simulink library "SUB_ECU_L4_MABX_HW_Interface"  (R2018a)
settings: Solver=VariableStepAuto  StartTime=0.0  StopTime=10.0  RelTol=1e-3
PostLoadFcn:
  | , if any(exist('dsrtsu_mdlpostloadfcn', 'file') == [2, 3, 6]), try dsrtsu_mdlpostloadfcn('Execute', bdroot); catch fprintf('Error in PostLoadFcn (dsrtsu_mdlpostloadfcn) for model "%s":\n %s\n', bdroot, lasterr); end, end,
undefined symbols (not defined in the file or in its folder): CANR_PROPB_REAX_3_13_CHANNEL_APV, CANR_PROPB_REAX_4_13_CHANNEL_APV, CANR_PROPB_XPR_1_50_CHANNEL_APV, ENUM_CAN_RX_T, ENUM_CAN_TX_T, ENUM_REAX_OPERATION_MODE_T, ENUM_SIGNAL_HEALTH_T, ENUM_XBR_CONTROL_MODE_T, ENUM_XBR_EBI_MODE_T, ENUM_XBR_PASS_THROUGH_ACTIVE_T, ENUM_XBR_PRIORITY_T, ENUM_XPR_INHIBIT_PARK_MANUAL_T, ENUM_XPR_INHIBIT_UNPARK_MANUAL_T, ENUM_XPR_PARK_MANUAL_T, ENUM_XPR_UNPARK_MANUAL_T, PROPB_REAX_1_E4_DES_POS_SIG_SRC_APV, PROPB_REAX_1_E4_DESIRED_OPMODE_APV, PROPB_REAX_1_E4_DESIRED_POSITION_APV, ptc_matlab_lib
libraries: PTC_MBDS_LIB x264, rtican x172, EmE_MBD_Blockset x39, simulink x34, $bdroot x16, rti1401lib_dio_type4 x8, simulink_need_slupdate x7, dsa_tcpip_lib x4, rti1401lib_adc_type4 x3, rtmapslib x3, rtitasklib x3
(part 1 of 51)
settings Model: DSRTSU_INTERNAL_RTI_VER=520  DSRTSU_INTERNAL_RTI_TYPE=rti1401  RTICANMMDATA=struct('GeneralSetupData',struct('modelroot','C:\data\svn\adv_adas_shared\trunk\Project_L4\src\ProjectLibrary','generalsettings',struct('filesettings',struct('destfolder',struct('Name','RTICANMM_FILES','Check',1),'buildfolder',struct('Name','.','Check',1),'AbsDestfolder',struct('Name','C:\data\svn\adv_adas_shared\trunk\Project_L4\src\ProjectLibrary\RTICANMM_FILES'),'AbsBuildfolder',struct('Name','C:\data\svn\adv_adas_shared\trunk\Project_L4\src\ProjectLibrary'))),'options',struct('addpaths',1,'rmpaths',1,'addtrcexclusion',logical(1),'cannavigator',struct('checkmonitoring',0),'show_usrtrc',0,'use_usrtrc',0),'advanced',struct('options',[1 1 1 1 1 1 1 1 1 1 1 1 1 1 1 1 1 1 1 1 1 1 1 1 1 1 1 1 1 1 1 1 1 1 1 1 1 1 1 1 1 1 1 1 1 1 1 1 1 1 1 1 1 1 1 1 1 1 1 1 1 1 1 1 1 1 1 1 1 1 1 1 1 1 1 1 1 1 1 1 1 1 1 1 1 1 1 1 1 1 1 1 1 1 1 1 1 1 1 1]),'MPSetup',{{}},'modelname','SUB_ECU_L4_MABX_HW_Interface','block','SUB_ECU_L4_MABX_HW_Interface'))  DSRTSU_INTERNAL_RTIFLEXRAYCONFIG=110  DSRTSU_INTERNAL_RTIFPGA=110  Creator=Chris.Balton  LastModifiedBy=Charles.Swart

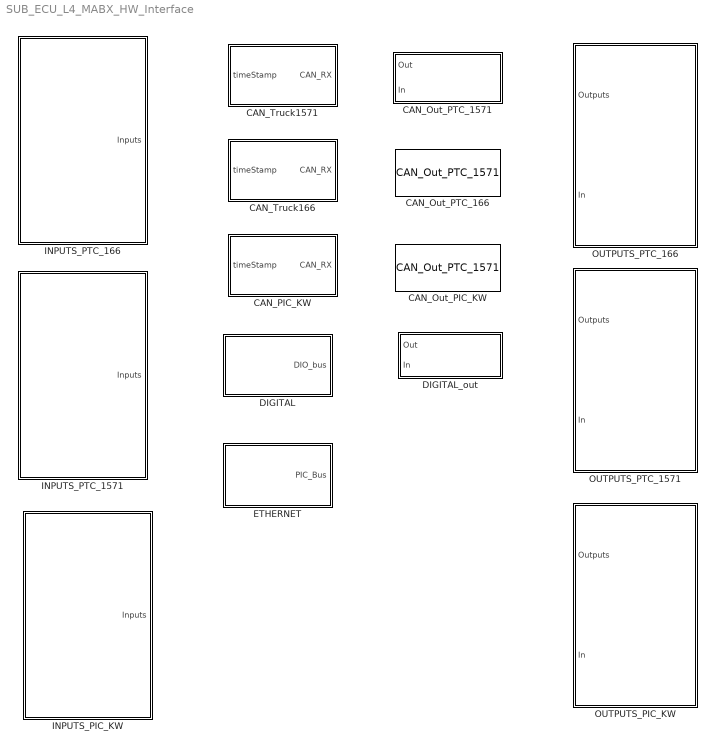
== system SUB_ECU_L4_MABX_HW_Interface ==
  CAN_Out_PIC_KW : $bdroot/CAN_Out_PTC_1571
  CAN_Out_PTC_1571 : Subsystem
  CAN_Out_PTC_166 : $bdroot/CAN_Out_PTC_1571
  CAN_PIC_KW : Subsystem
  CAN_Truck1571 : Subsystem
  CAN_Truck166 : Subsystem
  DIGITAL : Subsystem
  DIGITAL_out : Subsystem
  ETHERNET : Subsystem
  INPUTS_PIC_KW : Subsystem
  INPUTS_PTC_1571 : Subsystem
  INPUTS_PTC_166 : Subsystem
  OUTPUTS_PIC_KW : Subsystem
  OUTPUTS_PTC_1571 : Subsystem
  OUTPUTS_PTC_166 : Subsystem

== system SUB_ECU_L4_MABX_HW_Interface/CAN_Out_PTC_1571 ==
  Out : Inport
  In : Inport  Port=2
  CAN_TX_10000ms : Subsystem  TreatAsAtomicUnit=on  SystemSampleTime=10
  CAN_TX_1000ms : Subsystem  TreatAsAtomicUnit=on  SystemSampleTime=1
  CAN_TX_100ms : Subsystem  TreatAsAtomicUnit=on  SystemSampleTime=0.1
  CAN_TX_10ms : Subsystem  TreatAsAtomicUnit=on  SystemSampleTime=0.01
  CAN_TX_20ms : Subsystem  TreatAsAtomicUnit=on  SystemSampleTime=0.02
  CAN_TX_250ms : Subsystem  TreatAsAtomicUnit=on  SystemSampleTime=0.25
  CAN_TX_5000ms : Subsystem  TreatAsAtomicUnit=on  SystemSampleTime=5
  CAN_TX_50ms : Subsystem  TreatAsAtomicUnit=on  SystemSampleTime=0.05
  CAN_TX_BAM : Subsystem
  CAN_TX_VariableRate : Subsystem
  wires:
  In/1 -> CAN_TX_50ms/1(50msCAN), CAN_TX_1000ms/1(1000msCAN), CAN_TX_VariableRate/1(Feedthrough), CAN_TX_100ms/2(Feedthrough), CAN_TX_10ms/2(In)
  Out/1 -> CAN_TX_10ms/1(10msCAN), CAN_TX_20ms/1(20msCAN), CAN_TX_250ms/1(250msCAN), CAN_TX_5000ms/1(5000msCAN), CAN_TX_10000ms/1(10000msCAN), CAN_TX_100ms/1(100msCAN)
